simulink model "Noise"  (R2021a)
settings: Solver=VariableStepAuto  StartTime=0.0  StopTime=200  RelTol=1e-3
libraries: simulink x4
settings Model: Creator=templ  LastModifiedBy=templ
settings DataIOCC: ReturnWorkspaceOutputs=off

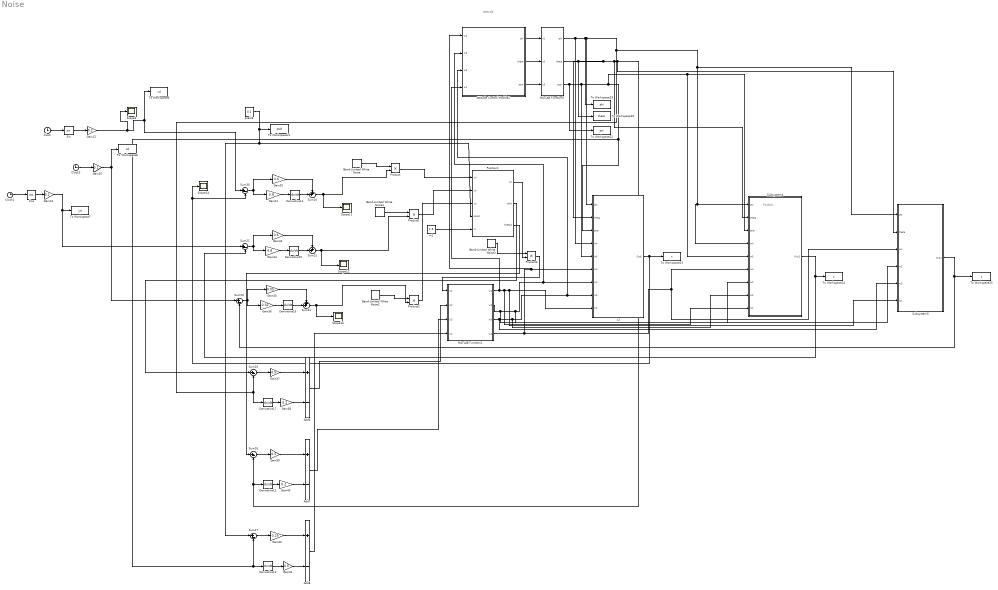
== system Noise ==
  note: Position
  note: Attitude
  Add6 : Sum  Inputs=+-
  Add7 : Sum  Inputs=+-
  Add8 : Sum  Inputs=+-
  Attitude Control Module2 : Subsystem
  Band-Limited White Noise{,1..3} (4 alike) : simulink/Sources/Band-Limited White Noise  Cov=[0.1]  Ts=0.1  seed=[23341]
  Clock : Clock
  Clock1 : Clock
  Clock3 : Clock
  Cos : Trigonometry  Operator=cos
  Derivative{12..17} (6 alike) : Derivative
  Gain{12..13,38,40} (4 alike) : Gain  Gain=0.2
  Gain15 : Gain  Gain=0.1
  Gain20 : Gain  Gain=0.6
  Gain21 : Gain  Gain=0.8
  Gain30 : Gain  Gain=0.25
  Gain31 : Gain  Gain=0.5
  Gain33 : Gain  Gain=0.6
  Gain34 : Gain  Gain=0.8
  Gain35 : Gain  Gain=0.05
  Gain36 : Gain  Gain=0.32
  Gain37 : Gain  Gain=0.5
  Gain39 : Gain  Gain=0.5
  MATLAB Function1 : MATLAB Function  TreatAsAtomicUnit=on
  MATLAB Function5 : MATLAB Function  TreatAsAtomicUnit=on
  Position1 : MATLAB Function  TreatAsAtomicUnit=on
  Product{,1..3} (4 alike) : Product
  Scope{3,11..14} (5 alike) : Scope
  Sin : Trigonometry
  Subsystem4 : Subsystem
  Subsystem5 : Subsystem
  Sum20 : Sum  Inputs=++|
  Sum{21,23,25..27,30} (6 alike) : Sum  Inputs=|+-
  Sum22 : Sum  Inputs=++|
  Sum24 : Sum  Inputs=++|
  To Workspace20 : ToWorkspace  VariableName=theta  SampleTime=-1
  To Workspace21 : ToWorkspace  VariableName=psid  SampleTime=-1
  To Workspace22 : ToWorkspace  VariableName=psi  SampleTime=-1
  To Workspace23 : ToWorkspace  VariableName=x  SampleTime=-1
  To Workspace24 : ToWorkspace  VariableName=y  SampleTime=-1
  To Workspace25 : ToWorkspace  VariableName=z  SampleTime=-1
  To Workspace29 : ToWorkspace  VariableName=phi  SampleTime=-1
  To Workspace6 : ToWorkspace  VariableName=xd  SampleTime=-1
  To Workspace7 : ToWorkspace  VariableName=yd  SampleTime=-1
  To Workspace8 : ToWorkspace  VariableName=zd  SampleTime=-1
  m1 : Constant  Value=1.5
  psaid3 : Constant  Value=0.2
  x2 : Subsystem
  wires:
  Subsystem4/1(Out1) -> Sum21/2, To Workspace24/1
  x2/1(Out1) -> Sum30/2, Scope14/1, To Workspace23/1
  MATLAB Function1/4(w4) -> Subsystem5/3(w4), Subsystem4/6(w4), Attitude Control Module2/1(w4), x2/6(w4)
  Attitude Control Module2/3(psai) -> MATLAB Function5/3(u3)
  Add7/1 -> MATLAB Function1/3(U3)
  Sum24/1 -> Scope13/1, Product2/2
  m1/1 -> Position1/5(m)
  Sum27/1 -> Gain30/1
  Gain30/1 -> Add8/1
  Gain37/1 -> Add6/1
  Gain34/1 -> Derivative15/1
  Derivative15/1 -> Sum22/2
  Derivative13/1 -> Gain31/1
  Attitude Control Module2/2(theta) -> MATLAB Function5/2(u2)
  Position1/2(phid) -> Sum25/1
  MATLAB Function1/1(w1) -> Attitude Control Module2/4(w1), Subsystem4/9(w1), Subsystem5/6(w1), x2/9(w1)
  Clock3/1 -> Gain15/1
  Gain33/1 -> Sum22/1
  Add8/1 -> MATLAB Function1/4(U4)
  Gain13/1 -> Sum21/1, To Workspace7/1
  Gain20/1 -> Sum20/1
  Gain36/1 -> Derivative16/1
  Subsystem5/1(Out1) -> Sum23/2, To Workspace25/1
  Add6/1 -> MATLAB Function1/2(U2)
  Sum20/1 -> Scope11/1, Product/2
  Sum25/1 -> Gain37/1
  Gain38/1 -> Add6/2
  MATLAB Function5/3(psai) -> To Workspace22/1, Subsystem4/5(In5), Subsystem4/3(psai), Sum27/2, Derivative13/1, x2/3(psai), x2/5(In5)
  Position1/3(thetad) -> Sum26/1
  Derivative12/1 -> Gain40/1
  psaid3/1 -> Sum27/1, Position1/4(psaid), To Workspace21/1
  MATLAB Function5/1(phi) -> x2/4(In4), To Workspace29/1, Derivative17/1, Sum25/2, Subsystem5/1(phi), Subsystem4/4(In4), Subsystem4/1(phi), x2/1(phi)
  Gain31/1 -> Add8/2
  Derivative17/1 -> Gain38/1
  Sum22/1 -> Scope12/1, Product1/2
  Gain35/1 -> Sum24/1
  Position1/1(U1) -> Product3/2
  Gain12/1 -> Scope3/1, To Workspace6/1, Sum30/1
  Sum23/1 -> Gain36/1, Gain35/1
  Derivative14/1 -> Sum20/2
  Sum26/1 -> Gain39/1
  Gain15/1 -> Sum23/1, To Workspace8/1
  Gain39/1 -> Add7/1
  Gain40/1 -> Add7/2
  MATLAB Function5/2(theta) -> To Workspace20/1, Sum26/2, Derivative12/1, Subsystem5/2(theta), Subsystem4/2(theta), x2/2(theta)
  Attitude Control Module2/1(phi) -> MATLAB Function5/1(u1)
  Gain21/1 -> Derivative14/1
  Sum30/1 -> Gain21/1, Gain20/1
  Sum21/1 -> Gain34/1, Gain33/1
  Derivative16/1 -> Sum24/2
  MATLAB Function1/2(w2) -> Subsystem5/4(w2), Subsystem4/7(w2), Attitude Control Module2/2(w2), x2/7(w2)
  MATLAB Function1/3(w3) -> Subsystem5/5(w3), Subsystem4/8(w3), Attitude Control Module2/3(w3), x2/8(w3)
  Band-Limited White Noise/1 -> Product/1
  Product/1 -> Position1/1(Ux)
  Band-Limited White Noise1/1 -> Product1/1
  Product1/1 -> Position1/2(Uy)
  Band-Limited White Noise2/1 -> Product2/1
  Product2/1 -> Position1/3(Uz)
  Band-Limited White Noise3/1 -> Product3/1
  Product3/1 -> MATLAB Function1/1(U1)
  Clock/1 -> Sin/1
  Sin/1 -> Gain12/1
  Clock1/1 -> Cos/1
  Cos/1 -> Gain13/1

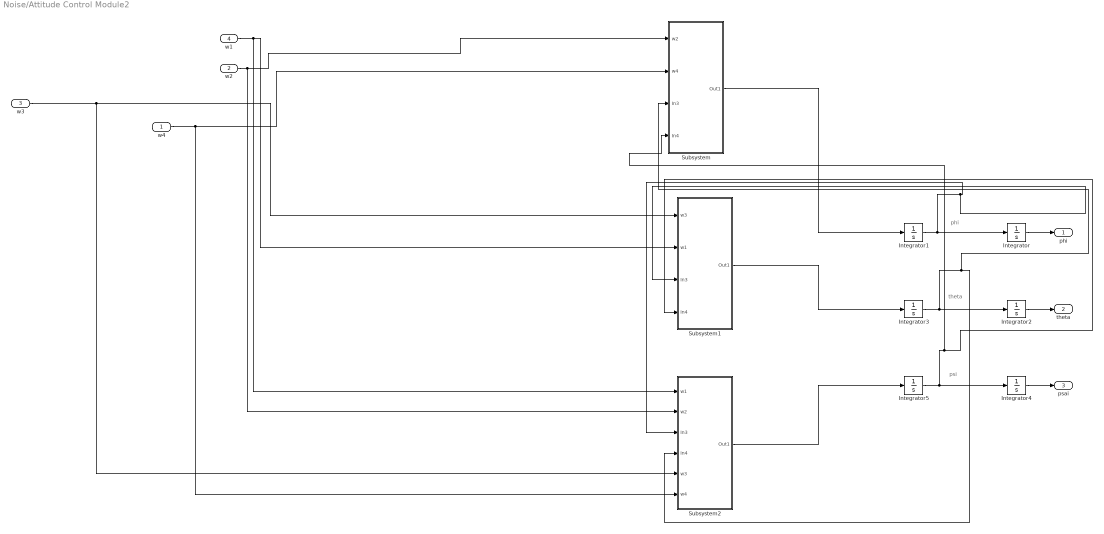
== system Noise/Attitude Control Module2 ==
  note: phi
  note: theta
  note: psi
  w4 : Inport
  w2 : Inport  Port=2
  w3 : Inport  Port=3
  w1 : Inport  Port=4
  Integrator{,1..5} (6 alike) : Integrator
  Subsystem : Subsystem
  Subsystem1 : Subsystem
  Subsystem2 : Subsystem
  phi : Outport  VectorParamsAs1DForOutWhenUnconnected=off
  theta : Outport  Port=2  VectorParamsAs1DForOutWhenUnconnected=off
  psai : Outport  Port=3  VectorParamsAs1DForOutWhenUnconnected=off
  wires:
  w2/1 -> Subsystem2/2(w2), Subsystem/1(w2)
  Subsystem/1(Out1) -> Integrator1/1
  Integrator3/1 -> Subsystem2/4(In4), Subsystem/3(In3), Integrator2/1
  Integrator1/1 -> Subsystem2/3(In3), Subsystem1/3(In3), Integrator/1
  Integrator5/1 -> Subsystem/4(In4), Subsystem1/4(In4), Integrator4/1
  w4/1 -> Subsystem2/6(w4), Subsystem/2(w4)
  Subsystem2/1(Out1) -> Integrator5/1
  w1/1 -> Subsystem2/1(w1), Subsystem1/2(w1)
  Integrator2/1 -> theta/1
  Integrator/1 -> phi/1
  Integrator4/1 -> psai/1
  Subsystem1/1(Out1) -> Integrator3/1
  w3/1 -> Subsystem2/5(w3), Subsystem1/1(w3)

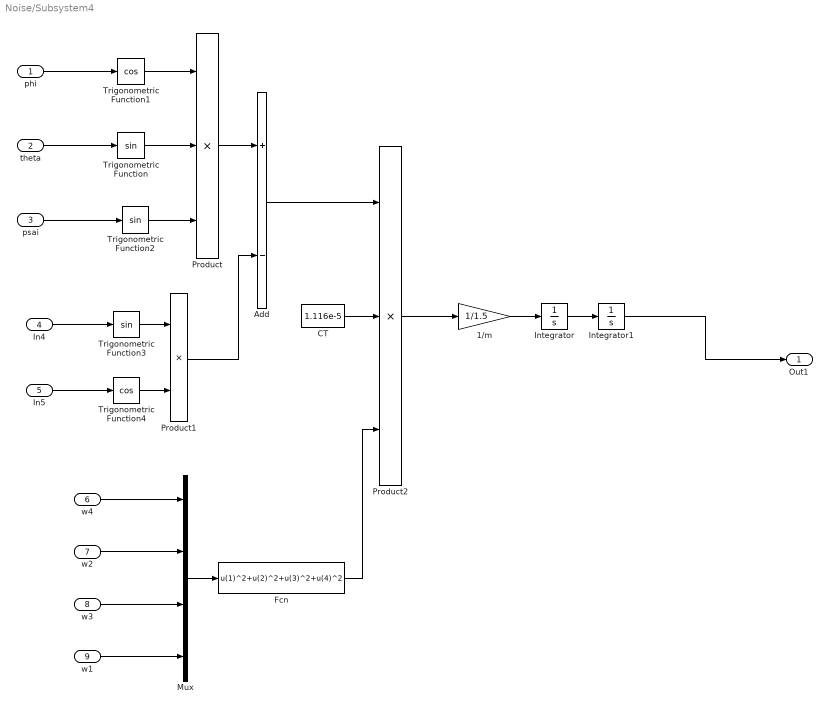
== system Noise/Subsystem4 ==
  phi : Inport
  theta : Inport  Port=2
  psai : Inport  Port=3
  In4 : Inport  Port=4
  In5 : Inport  Port=5
  w4 : Inport  Port=6
  w2 : Inport  Port=7
  w3 : Inport  Port=8
  w1 : Inport  Port=9
  1/m : Gain  Gain=1/1.5
  Add : Sum  Inputs=+-
  CT : Constant  Value=1.116e-5
  Fcn : Fcn  Expr=u(1)^2+u(2)^2+u(3)^2+u(4)^2
  Integrator : Integrator
  Integrator1 : Integrator
  Mux : Mux
  Product : Product  Inputs=3
  Product1 : Product
  Product2 : Product  Inputs=3
  Trigonometric Function : Trigonometry
  Trigonometric Function1 : Trigonometry  Operator=cos
  Trigonometric Function2 : Trigonometry
  Trigonometric Function3 : Trigonometry
  Trigonometric Function4 : Trigonometry  Operator=cos
  Out1 : Outport  VectorParamsAs1DForOutWhenUnconnected=off
  wires:
  Mux/1 -> Fcn/1
  Product2/1 -> 1/m/1
  Fcn/1 -> Product2/3
  CT/1 -> Product2/2
  Trigonometric Function2/1 -> Product/3
  Trigonometric Function/1 -> Product/2
  Trigonometric Function3/1 -> Product1/1
  Product1/1 -> Add/2
  Product/1 -> Add/1
  Add/1 -> Product2/1
  In4/1 -> Trigonometric Function3/1
  Trigonometric Function1/1 -> Product/1
  Integrator/1 -> Integrator1/1
  w3/1 -> Mux/3
  Trigonometric Function4/1 -> Product1/2
  1/m/1 -> Integrator/1
  Integrator1/1 -> Out1/1
  w1/1 -> Mux/4
  phi/1 -> Trigonometric Function1/1
  w4/1 -> Mux/1
  In5/1 -> Trigonometric Function4/1
  w2/1 -> Mux/2
  psai/1 -> Trigonometric Function2/1
  theta/1 -> Trigonometric Function/1

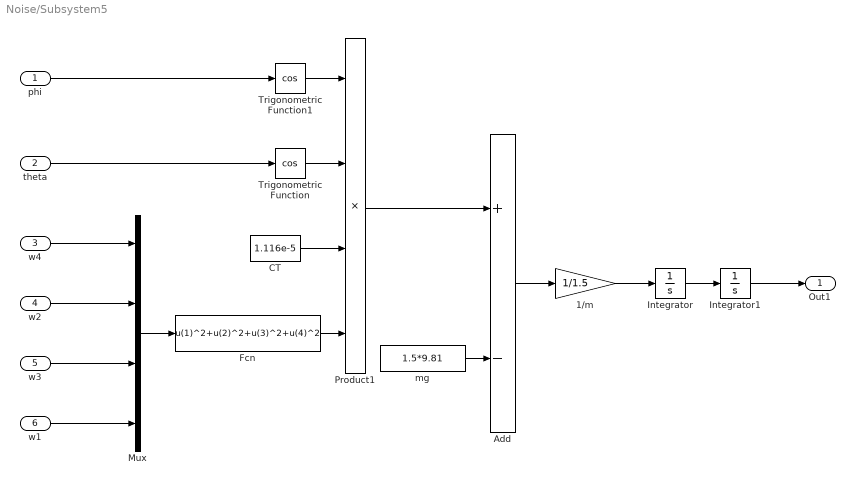
== system Noise/Subsystem5 ==
  phi : Inport
  theta : Inport  Port=2
  w4 : Inport  Port=3
  w2 : Inport  Port=4
  w3 : Inport  Port=5
  w1 : Inport  Port=6
  1/m : Gain  Gain=1/1.5
  Add : Sum  Inputs=+-
  CT : Constant  Value=1.116e-5
  Fcn : Fcn  Expr=u(1)^2+u(2)^2+u(3)^2+u(4)^2
  Integrator : Integrator
  Integrator1 : Integrator
  Mux : Mux
  Product1 : Product  Inputs=4
  Trigonometric Function : Trigonometry  Operator=cos
  Trigonometric Function1 : Trigonometry  Operator=cos
  mg : Constant  Value=1.5*9.81
  Out1 : Outport  VectorParamsAs1DForOutWhenUnconnected=off
  wires:
  Trigonometric Function1/1 -> Product1/1
  Integrator/1 -> Integrator1/1
  Fcn/1 -> Product1/4
  mg/1 -> Add/2
  CT/1 -> Product1/3
  Add/1 -> 1/m/1
  Mux/1 -> Fcn/1
  theta/1 -> Trigonometric Function/1
  1/m/1 -> Integrator/1
  Trigonometric Function/1 -> Product1/2
  Product1/1 -> Add/1
  w2/1 -> Mux/2
  Integrator1/1 -> Out1/1
  w3/1 -> Mux/3
  w4/1 -> Mux/1
  w1/1 -> Mux/4
  phi/1 -> Trigonometric Function1/1

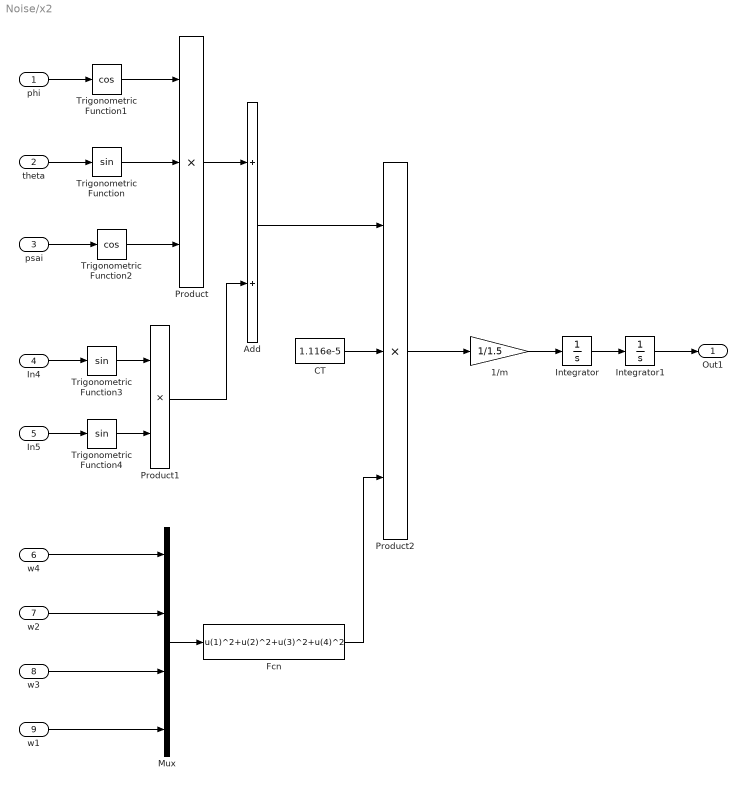
== system Noise/x2 ==
  phi : Inport
  theta : Inport  Port=2
  psai : Inport  Port=3
  In4 : Inport  Port=4
  In5 : Inport  Port=5
  w4 : Inport  Port=6
  w2 : Inport  Port=7
  w3 : Inport  Port=8
  w1 : Inport  Port=9
  1/m : Gain  Gain=1/1.5
  Add : Sum
  CT : Constant  Value=1.116e-5
  Fcn : Fcn  Expr=u(1)^2+u(2)^2+u(3)^2+u(4)^2
  Integrator : Integrator
  Integrator1 : Integrator
  Mux : Mux
  Product : Product  Inputs=3
  Product1 : Product
  Product2 : Product  Inputs=3
  Trigonometric Function : Trigonometry
  Trigonometric Function1 : Trigonometry  Operator=cos
  Trigonometric Function2 : Trigonometry  Operator=cos
  Trigonometric Function3 : Trigonometry
  Trigonometric Function4 : Trigonometry
  Out1 : Outport  VectorParamsAs1DForOutWhenUnconnected=off
  wires:
  w3/1 -> Mux/3
  Integrator1/1 -> Out1/1
  1/m/1 -> Integrator/1
  Trigonometric Function4/1 -> Product1/2
  Integrator/1 -> Integrator1/1
  w2/1 -> Mux/2
  Add/1 -> Product2/1
  Product1/1 -> Add/2
  Product/1 -> Add/1
  In4/1 -> Trigonometric Function3/1
  Fcn/1 -> Product2/3
  Trigonometric Function1/1 -> Product/1
  theta/1 -> Trigonometric Function/1
  Trigonometric Function/1 -> Product/2
  Trigonometric Function2/1 -> Product/3
  Trigonometric Function3/1 -> Product1/1
  CT/1 -> Product2/2
  phi/1 -> Trigonometric Function1/1
  Product2/1 -> 1/m/1
  psai/1 -> Trigonometric Function2/1
  Mux/1 -> Fcn/1
  w4/1 -> Mux/1
  In5/1 -> Trigonometric Function4/1
  w1/1 -> Mux/4

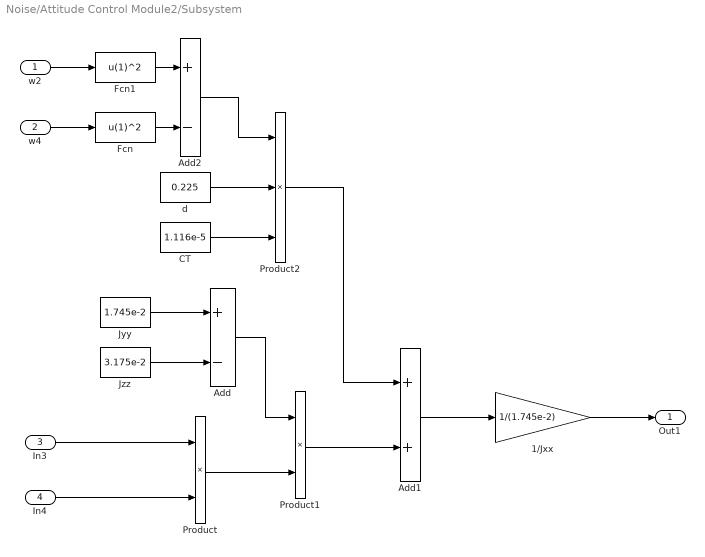
== system Noise/Attitude Control Module2/Subsystem ==
  w2 : Inport
  w4 : Inport  Port=2
  In3 : Inport  Port=3
  In4 : Inport  Port=4
  1/Jxx : Gain  Gain=1/(1.745e-2)
  Add : Sum  Inputs=+-
  Add1 : Sum
  Add2 : Sum  Inputs=+-
  CT : Constant  Value=1.116e-5
  Fcn : Fcn  Expr=u(1)^2
  Fcn1 : Fcn  Expr=u(1)^2
  Jyy : Constant  Value=1.745e-2
  "Jzz " : Constant  Value=3.175e-2
  Product : Product
  Product1 : Product
  Product2 : Product  Inputs=3
  d : Constant  Value=0.225
  Out1 : Outport  VectorParamsAs1DForOutWhenUnconnected=off
  wires:
  Product2/1 -> Add1/1
  Fcn/1 -> Add2/2
  CT/1 -> Product2/3
  "Jzz "/1 -> Add/2
  Add1/1 -> 1/Jxx/1
  Fcn1/1 -> Add2/1
  Add2/1 -> Product2/1
  Product1/1 -> Add1/2
  Product/1 -> Product1/2
  d/1 -> Product2/2
  In4/1 -> Product/2
  Jyy/1 -> Add/1
  w4/1 -> Fcn/1
  Add/1 -> Product1/1
  1/Jxx/1 -> Out1/1
  w2/1 -> Fcn1/1
  In3/1 -> Product/1

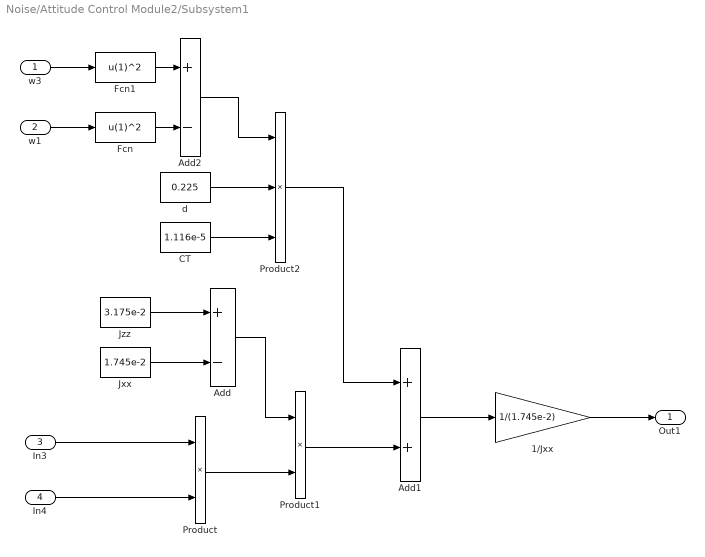
== system Noise/Attitude Control Module2/Subsystem1 ==
  w3 : Inport
  w1 : Inport  Port=2
  In3 : Inport  Port=3
  In4 : Inport  Port=4
  1/Jxx : Gain  Gain=1/(1.745e-2)
  Add : Sum  Inputs=+-
  Add1 : Sum
  Add2 : Sum  Inputs=+-
  CT : Constant  Value=1.116e-5
  Fcn : Fcn  Expr=u(1)^2
  Fcn1 : Fcn  Expr=u(1)^2
  Jxx : Constant  Value=1.745e-2
  Jzz : Constant  Value=3.175e-2
  Product : Product
  Product1 : Product
  Product2 : Product  Inputs=3
  d : Constant  Value=0.225
  Out1 : Outport  VectorParamsAs1DForOutWhenUnconnected=off
  wires:
  Product2/1 -> Add1/1
  Fcn/1 -> Add2/2
  CT/1 -> Product2/3
  Jxx/1 -> Add/2
  Add1/1 -> 1/Jxx/1
  Fcn1/1 -> Add2/1
  Add2/1 -> Product2/1
  Product1/1 -> Add1/2
  Product/1 -> Product1/2
  d/1 -> Product2/2
  In4/1 -> Product/2
  Jzz/1 -> Add/1
  w1/1 -> Fcn/1
  Add/1 -> Product1/1
  1/Jxx/1 -> Out1/1
  w3/1 -> Fcn1/1
  In3/1 -> Product/1

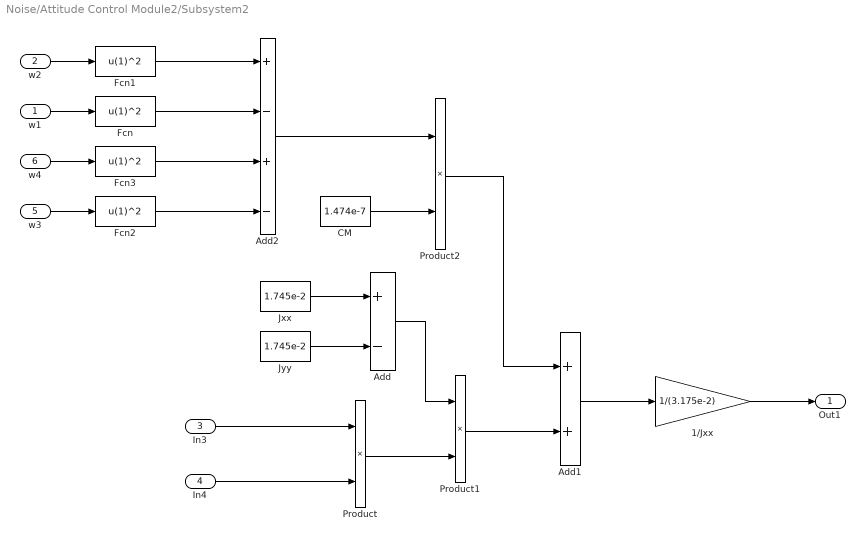
== system Noise/Attitude Control Module2/Subsystem2 ==
  w1 : Inport
  w2 : Inport  Port=2
  In3 : Inport  Port=3
  In4 : Inport  Port=4
  w3 : Inport  Port=5
  w4 : Inport  Port=6
  1/Jxx : Gain  Gain=1/(3.175e-2)
  Add : Sum  Inputs=+-
  Add1 : Sum
  Add2 : Sum  Inputs=+-+-
  CM : Constant  Value=1.474e-7
  Fcn{,1..3} (4 alike) : Fcn  Expr=u(1)^2
  Jxx : Constant  Value=1.745e-2
  Jyy : Constant  Value=1.745e-2
  Product : Product
  Product1 : Product
  Product2 : Product
  Out1 : Outport  VectorParamsAs1DForOutWhenUnconnected=off
  wires:
  Product2/1 -> Add1/1
  CM/1 -> Product2/2
  Jyy/1 -> Add/2
  Add1/1 -> 1/Jxx/1
  Add2/1 -> Product2/1
  Product1/1 -> Add1/2
  Product/1 -> Product1/2
  In4/1 -> Product/2
  Jxx/1 -> Add/1
  Add/1 -> Product1/1
  1/Jxx/1 -> Out1/1
  In3/1 -> Product/1
  Fcn1/1 -> Add2/1
  Fcn/1 -> Add2/2
  Fcn3/1 -> Add2/3
  Fcn2/1 -> Add2/4
  w2/1 -> Fcn1/1
  w4/1 -> Fcn3/1
  w1/1 -> Fcn/1
  w3/1 -> Fcn2/1

== matlab function Noise/MATLAB Function5 ==
  data: u1 input; phi output; u2 input; u3 input; theta output; psai output
function [phi, theta, psai] = fcn(u1, u2, u3)

    phi = rem(u1,2*pi);
    theta = rem(u2,2*pi);
    psai = rem(u3,2*pi);
end

== matlab function Noise/MATLAB Function1 ==
  data: U1 input; w1 output; U2 input; U3 input; U4 input; w2 output; w3 output; w4 output
function [w1,w2,w3,w4] = fcn(U1,U2,U3,U4)
    CT = 1.116e-5; dCT = 0.225*CT;
    matrixA = [CT,CT,CT,CT;0,CT,0,-CT;-CT,0,CT,0;-dCT,dCT,-dCT,dCT];
    w_2 = inv(matrixA)*[U1,U2,U3,U4]';
    w1 = sqrt(abs(w_2(1))); w2 = sqrt(abs(w_2(2)));
    w3 = sqrt(abs(w_2(3))); w4 = sqrt(abs(w_2(4)));
end

== matlab function Noise/Position1 ==
  data: Ux input; U1 output; Uy input; Uz input; psaid input; m input; phid output; thetad output
function [U1,phid,thetad] = fcn(Ux,Uy,Uz,psaid,m)
    U1 = m*sqrt(Ux^2+Uy^2+(Uz+9.81)^2);
    phid = asin((Ux*sin(psaid)-Uy*cos(psaid))*m/U1);
%     thetad = asin((Ux*m-U1*sin(psaid)*sin(phid))/(U1*cos(psaid)*cos(phid)));
thetad=atan((Ux*cos(psaid)+Uy*sin(psaid))/(Uz+9.81));
end
